simulink model "model_plusacc_2018b"  (R2018a)
settings: Solver=FixedStepAuto  StartTime=0.0  StopTime=10000  FixedStep=1  RelTol=1e-3
values from neighbouring files (symbols this model uses):
  r_start = [aux_p(1:3) r_0 aux_p(4:end)]    [Five_chasers_init.m]
  v_start = [aux_v(1:3) v_0 aux_v(4:end)]    [Five_chasers_init.m]
settings Model: Creator=Benny Rievers  LastModifiedBy=Riya Bhattacharjee

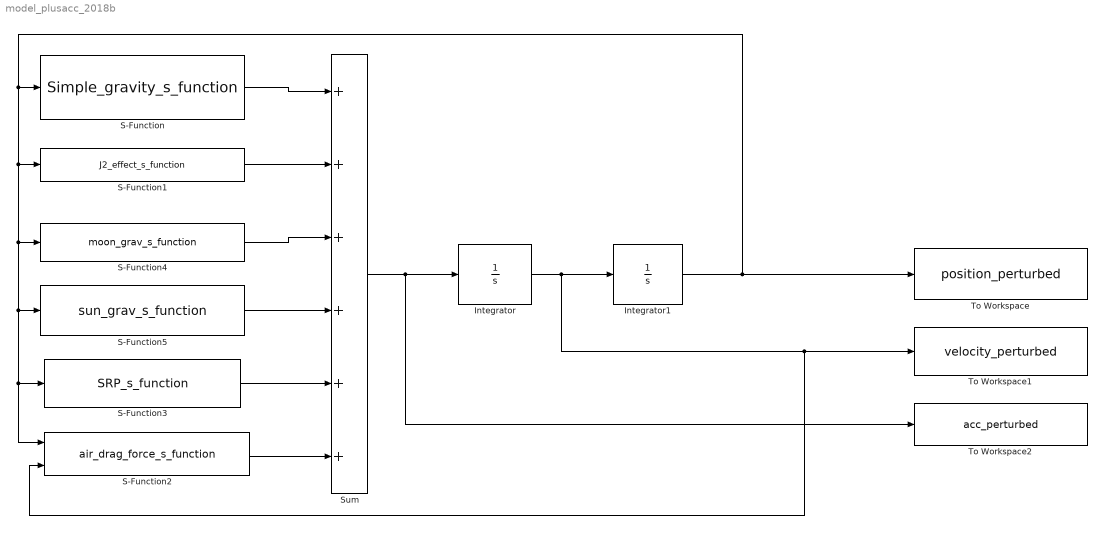
== system model_plusacc_2018b ==
  Integrator : Integrator  InitialCondition=v_start
  Integrator1 : Integrator  InitialCondition=r_start
  S-Function : S-Function  FunctionName=Simple_gravity_s_function  SFunctionDeploymentMode=off  EnableBusSupport=off
  S-Function1 : S-Function  FunctionName=J2_effect_s_function  SFunctionDeploymentMode=off  EnableBusSupport=off
  S-Function2 : S-Function  FunctionName=air_drag_force_s_function  SFunctionDeploymentMode=off  EnableBusSupport=off
  S-Function3 : S-Function  FunctionName=SRP_s_function  SFunctionDeploymentMode=off  EnableBusSupport=off
  S-Function4 : S-Function  FunctionName=moon_grav_s_function  SFunctionDeploymentMode=off  EnableBusSupport=off
  S-Function5 : S-Function  FunctionName=sun_grav_s_function  SFunctionDeploymentMode=off  EnableBusSupport=off
  Sum : Sum  Inputs=++++++  InputSameDT=on
  To Workspace : ToWorkspace  VariableName=position_perturbed  SampleTime=-1
  To Workspace1 : ToWorkspace  VariableName=velocity_perturbed  SampleTime=-1
  To Workspace2 : ToWorkspace  VariableName=acc_perturbed  SampleTime=-1
  wires:
  Integrator/1 -> S-Function2/2, To Workspace1/1, Integrator1/1
  Sum/1 -> To Workspace2/1, Integrator/1
  Integrator1/1 -> To Workspace/1, S-Function2/1, S-Function3/1, S-Function5/1, S-Function4/1, S-Function1/1, S-Function/1
  S-Function4/1 -> Sum/3
  S-Function/1 -> Sum/1
  S-Function1/1 -> Sum/2
  S-Function5/1 -> Sum/4
  S-Function3/1 -> Sum/5
  S-Function2/1 -> Sum/6
